simulink model "ex3"  (R2025b)
settings: Solver=VariableStepAuto  StartTime=0.0  StopTime=10.0  RelTol=1e-3
settings Model: Creator=vladl  LastModifiedBy=vladl

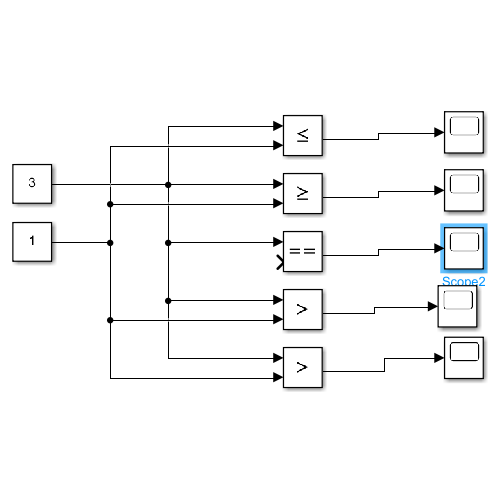
[thumbnail: Simulink's stored preview of the top-level diagram]
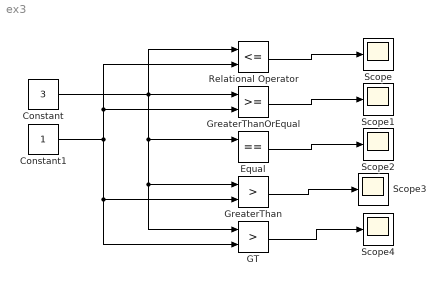
== system ex3 ==
  Constant : Constant  Value=3
  Constant1 : Constant
  Equal : RelationalOperator  Operator===  OutDataTypeStr=boolean  RndMeth=Simplest  InputSameDT=off
  GT : RelationalOperator  Operator=>  OutDataTypeStr=boolean  RndMeth=Simplest  InputSameDT=off
  GreaterThan : RelationalOperator  Operator=>  OutDataTypeStr=boolean  RndMeth=Simplest  InputSameDT=off
  GreaterThanOrEqual : RelationalOperator  OutDataTypeStr=boolean  RndMeth=Simplest  InputSameDT=off
  Relational Operator : RelationalOperator  Operator=<=  OutDataTypeStr=boolean  RndMeth=Simplest  InputSameDT=off
  Scope{,1..4} (5 alike) : Scope
      Scope settings: ActiveDisplayYMinimum=-1  ActiveDisplayYMaximum=1
      Scope1 settings: ActiveDisplayYMinimum=0.9  ActiveDisplayYMaximum=1.1
      Scope2 settings: ActiveDisplayYMinimum=-1  ActiveDisplayYMaximum=1  DataLoggingVariableName=ScopeData2
      Scope3 settings: DataLoggingVariableName=ScopeData3
      Scope4 settings: DataLoggingVariableName=ScopeData4
  wires:
  Constant/1 -> GT/1, GreaterThan/1, Equal/1, GreaterThanOrEqual/1, Relational Operator/1
  Constant1/1 -> GT/2, GreaterThan/2, GreaterThanOrEqual/2, Relational Operator/2
  Relational Operator/1 -> Scope/1
  GreaterThanOrEqual/1 -> Scope1/1
  Equal/1 -> Scope2/1
  GreaterThan/1 -> Scope3/1
  GT/1 -> Scope4/1
